simulink model "heading_model_controlled"  (Simulink 8.3)
settings: Solver=ode45  StartTime=tstart  StopTime=tstop  RelTol=1e-3
values from neighbouring files (symbols this model uses):
  c_ss = lsqcurvefit(p, c_0, r_tests, d_c_tests)    [run_task_1_3.m]
  K = -0.041    [run_task_1_3.m]
  psi_d = deg2rad(18)    [run_task_1_3.m]
  T = 80    [run_task_1_3.m]
  tsamp = 10    [run_task_1_3.m]
undefined symbols (not defined in the file or in its folder): K_d
settings Model: Creator=christh  LastModifiedBy=Hwk  ExtModeAutoUpdateStatusClock=off
settings OptimizationCC: ExpressionDepthLimit=2147483647  InitFltsAndDblsToZero=on
settings DebuggingCC: FcnCallInpInsideContextMsg=UseLocalSettings

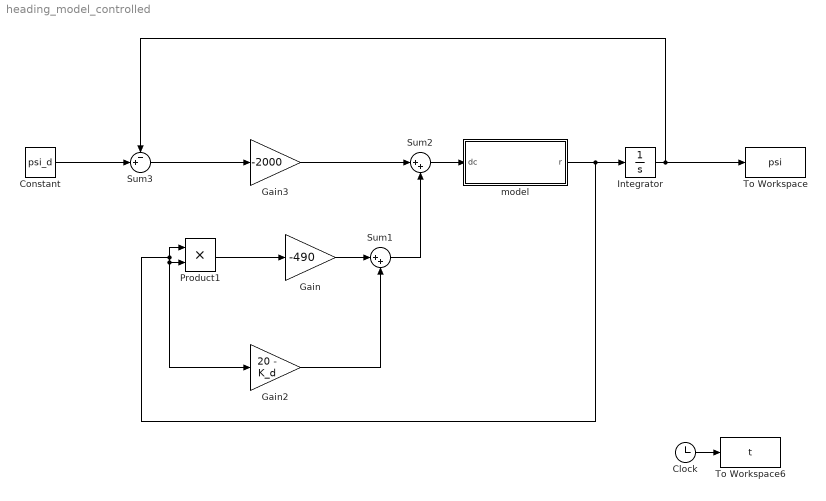
== system heading_model_controlled ==
  Clock : Clock
  Constant : Constant  Value=psi_d
  Gain : Gain  Gain=-490
  Gain2 : Gain  Gain=20 - K_d
  Gain3 : Gain  Gain=-2000
  Integrator : Integrator
  Product1 : Product
  Sum1 : Sum  Inputs=|++
  Sum2 : Sum  Inputs=|++
  Sum3 : Sum  Inputs=-+|
  To Workspace : ToWorkspace  VariableName=psi  SampleTime=tsamp
  To Workspace6 : ToWorkspace  VariableName=t  SampleTime=tsamp
  model : Subsystem
  wires:
  model/1(r) -> Product1/1, Gain2/1, Product1/2, Integrator/1
  Product1/1 -> Gain/1
  Gain2/1 -> Sum1/2
  Integrator/1 -> To Workspace/1, Sum3/1
  Sum1/1 -> Sum2/2
  Sum2/1 -> model/1(dc)
  Constant/1 -> Sum3/2
  Sum3/1 -> Gain3/1
  Gain3/1 -> Sum2/1
  Gain/1 -> Sum1/1
  Clock/1 -> To Workspace6/1

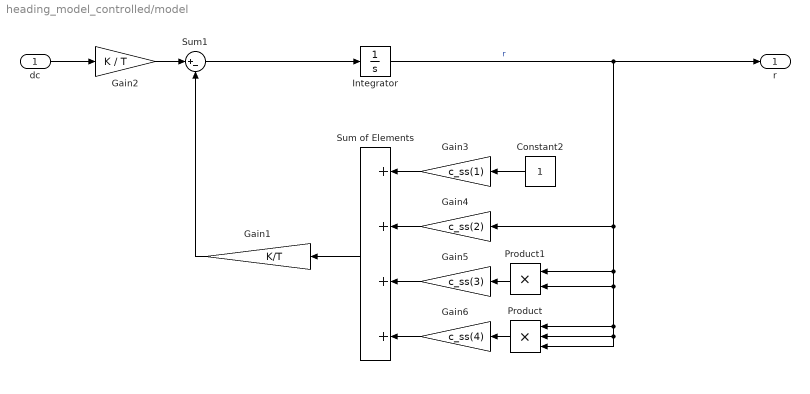
== system heading_model_controlled/model ==
  dc : Inport
  Constant2 : Constant
  Gain1 : Gain  Gain=K/T
  Gain2 : Gain  Gain=K / T
  Gain3 : Gain  Gain=c_ss(1)
  Gain4 : Gain  Gain=c_ss(2)
  Gain5 : Gain  Gain=c_ss(3)
  Gain6 : Gain  Gain=c_ss(4)
  Integrator : Integrator
  Product : Product  Inputs=3
  Product1 : Product
  Sum of Elements : Sum  Inputs=4
  Sum1 : Sum  Inputs=|+-
  r : Outport
  wires:
  Sum1/1 -> Integrator/1
  Gain1/1 -> Sum1/2
  dc/1 -> Gain2/1
  Gain2/1 -> Sum1/1
  Sum of Elements/1 -> Gain1/1
  Gain4/1 -> Sum of Elements/2
  Gain5/1 -> Sum of Elements/3
  Gain6/1 -> Sum of Elements/4
  Gain3/1 -> Sum of Elements/1
  Integrator/1 -> r/1, Gain4/1, Product/3, Product/2, Product/1, Product1/2, Product1/1  "r"
  Constant2/1 -> Gain3/1
  Product1/1 -> Gain5/1
  Product/1 -> Gain6/1
